simulink model "MiL_BMS_Bat"  (Simulink 7.8)
settings: Solver=ode1  SolverMode=SingleTasking  StartTime=0.0  StopTime=4000  FixedStep=0.01  RelTol=1e-3
PreLoadFcn:
  | Init_file_Bat;
values from neighbouring files (symbols this model uses):
  C_diff = 5000    [Init_file_Bat.m]
  ChargeCurrent = 5    [Init_file_Bat.m]
  ChargeSwitch = 1    [Init_file_Bat.m]
  delta_max_v_cell = 1    [Init_file_Bat.m]
  DischargeCurrent = -5    [Init_file_Bat.m]
  I_max_line = int32(10000)    [Init_file_Bat.m]
  I_min_line = int32(-10000)    [Init_file_Bat.m]
  n_cells = 12    [Init_file_Bat.m]
  poles_soc = polyfit(SoC_table, OCV_table,4)    [Init_file_Bat.m]
  Q_0 = 36000*ones(1,12)    [Init_file_Bat.m]
  R_balance = 10*ones(1,12)    [Init_file_Bat.m]
  R_ct = 3.2*10^-3    (= 0.0032)    [Init_file_Bat.m]
  R_diff = 4*10^-3    (= 0.004)    [Init_file_Bat.m]
  R_i = 2*10^-3    (= 0.002)    [Init_file_Bat.m]
  SoC_init_cells = 0.8*ones(1,12)    [Init_file_Bat.m]
  T_cells = 20*ones(1,12)    [Init_file_Bat.m]
  T_max_cell = uint16(373)    [Init_file_Bat.m]
  T_min_cell = uint16(273)    [Init_file_Bat.m]
  Ts = 10*10^-3    (= 0.01)    [Init_file_Bat.m]
  V_max_bat = uint16(49080)    [Init_file_Bat.m]
  V_max_cell = uint16(4090)    [Init_file_Bat.m]
  V_min_bat = uint16(36000)    [Init_file_Bat.m]
  V_min_cell = uint16(2800)    [Init_file_Bat.m]
undefined symbols (not defined in the file or in its folder): DiscIntNeverNeededParam, OCV_table, sigbuilder_block, SoC_table
settings Model: Creator=Schmidt  LastModifiedBy=user
settings DebuggingCC: FcnCallInpInsideContextMsg=Use local settings
settings RTWCC: SystemTargetFile=lcrt.tlc  TemplateMakefile=lcrt_default_tmf  Description=LABCAR Real-Time Target  ProcessScript=lcrt_make_rtw_hook
settings STFCustomTargetCC: ModelReferenceCompliant=off  SystemTargetFile=lcrt.tlc

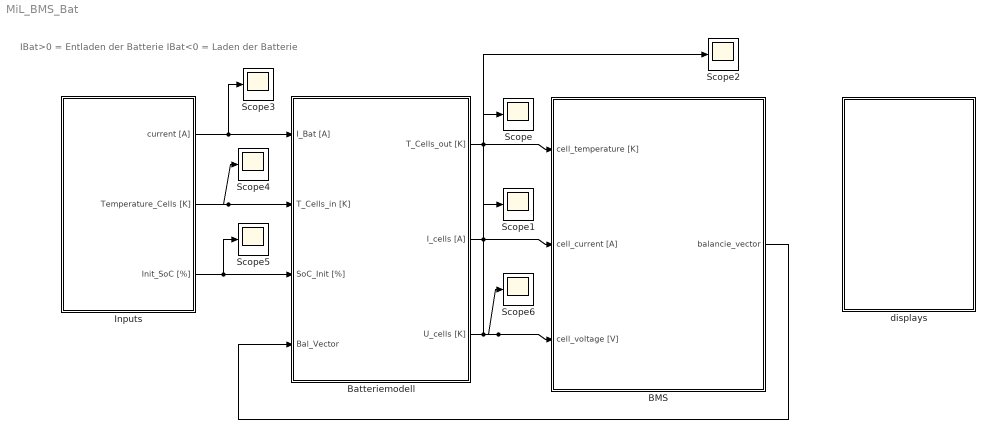
== system MiL_BMS_Bat ==
  note: IBat>0 = Entladen der Batterie
      | IBat<0 = Laden der Batterie
  BMS : Subsystem
  Batteriemodell : Subsystem
  Inputs : Subsystem
  Scope{,1..6} (7 alike) : Scope
      Scope settings: YMin=20  YMax=20  SaveName=ScopeData19
      Scope1 settings: YMin=-10  YMax=-10  SaveName=ScopeData20
      Scope2 settings: SaveName=ScopeData21
      Scope3 settings: YMin=-10  YMax=-10  SaveName=ScopeData22
      Scope4 settings: SaveName=ScopeData23
      Scope5 settings: SaveName=ScopeData24
      Scope6 settings: YMin=3.38  YMax=3.46  SaveName=ScopeData25
  displays : Subsystem
  wires:
  Batteriemodell/1(T_Cells_out [K]) -> BMS/1(cell_temperature [K]), Scope/1
  Inputs/1(current [A]) -> Batteriemodell/1(I_Bat [A]), Scope3/1
  Inputs/2(Temperature_Cells [K]) -> Batteriemodell/2(T_Cells_in [K]), Scope4/1
  Inputs/3(Init_SoC [%]) -> Batteriemodell/3(SoC_Init [%]), Scope5/1
  Batteriemodell/3(U_cells [K]) -> Scope2/1, BMS/3(cell_voltage [V]), Scope6/1
  Batteriemodell/2(I_cells [A]) -> BMS/2(cell_current [A]), Scope1/1
  BMS/1(balancie_vector) -> Batteriemodell/4(Bal_Vector)

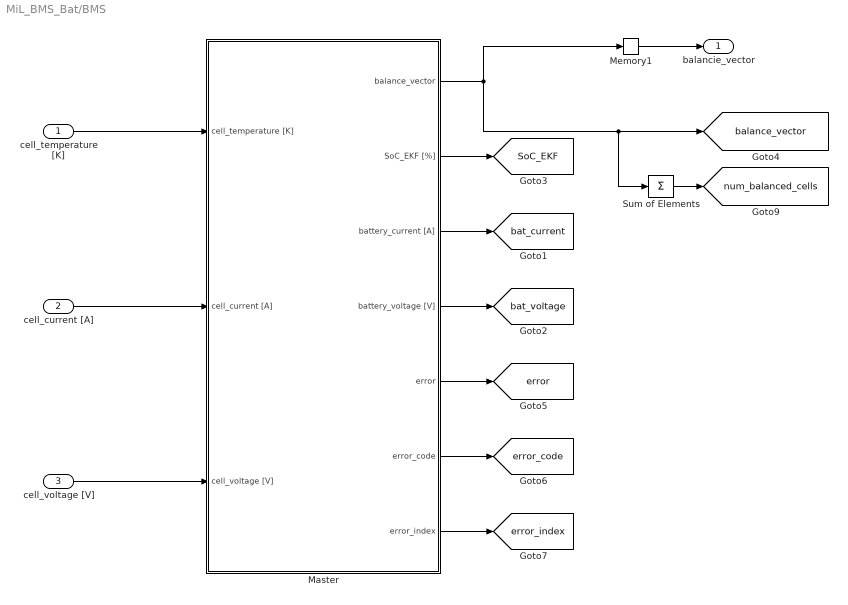
== system MiL_BMS_Bat/BMS ==
  cell_temperature [K] : Inport
  cell_current [A] : Inport  Port=2
  cell_voltage [V] : Inport  Port=3
  Master : Subsystem
  Memory1 : Memory
  Sum of Elements : Sum  Inputs=+
  balancie_vector : Outport
  tag scope: SoC_EKF=global, balance_vector=global, bat_current=global, bat_voltage=global, error=global, error_code=global, error_index=global, num_balanced_cells=global
  wires:
  Memory1/1 -> balancie_vector/1
  cell_temperature [K]/1 -> Master/1(cell_temperature [K])
  cell_voltage [V]/1 -> Master/3(cell_voltage [V])
  cell_current [A]/1 -> Master/2(cell_current [A])
  Master/2(SoC_EKF [%]) -> [SoC_EKF]
  Master/5(error) -> [error]
  Master/6(error_code) -> [error_code]
  Master/7(error_index) -> [error_index]
  Master/1(balance_vector) -> [balance_vector], Sum of Elements/1, Memory1/1
  Master/3(battery_current [A]) -> [bat_current]
  Master/4(battery_voltage [V]) -> [bat_voltage]
  Sum of Elements/1 -> [num_balanced_cells]

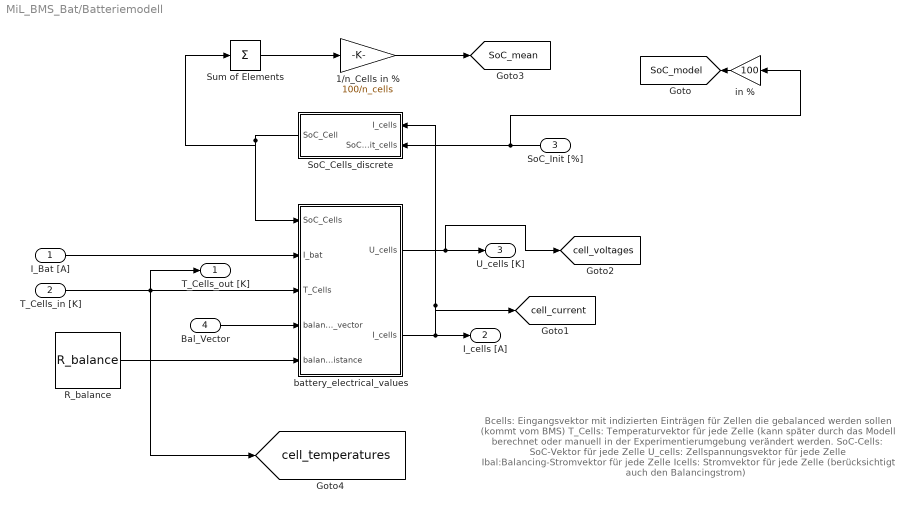
== system MiL_BMS_Bat/Batteriemodell ==
  note: Bcells: Eingangsvektor mit indizierten Einträgen
      | für Zellen die gebalanced werden sollen
      | (kommt vom BMS)
      |
      | T_Cells: Temperaturvektor für jede Zelle (kann später
      | durch das Modell berechnet oder manuell in der
      | Experimentierumgebung verändert werden.
      |
      | SoC-Cells: SoC-Vektor für jede Zelle
      |
      | U_cells: Zellspannungsvektor für jede Zelle
      |
      | Ibal:Balancing-Stromvektor für jede Zelle
      |
      | Icells: Stromvektor für jede Zelle (berücksichtigt auch
      | den Balancingstrom)
  I_Bat [A] : Inport
  T_Cells_in [K] : Inport  Port=2
  SoC_Init [%] : Inport  Port=3
  Bal_Vector : Inport  Port=4
  1/n_Cells in % : Gain  Gain=100/n_cells
  R_balance : Constant  Value=R_balance
  SoC_Cells_discrete : Subsystem
  Sum of Elements : Sum  Inputs=+
  battery_electrical_values : Subsystem
  in % : Gain  Gain=100
  T_Cells_out [K] : Outport
  I_cells [A] : Outport  Port=2
  U_cells [K] : Outport  Port=3
  tag scope: SoC_mean=global, SoC_model=global, cell_current=global, cell_temperatures=global, cell_voltages=global
  wires:
  in %/1 -> [SoC_model]
  Sum of Elements/1 -> 1/n_Cells in %/1
  1/n_Cells in %/1 -> [SoC_mean]
  SoC_Init [%]/1 -> SoC_Cells_discrete/2(SoC_init_cells), in %/1
  battery_electrical_values/2(I_cells) -> I_cells [A]/1, SoC_Cells_discrete/1(I_cells), [cell_current]
  SoC_Cells_discrete/1(SoC_Cell) -> battery_electrical_values/1(SoC_Cells), Sum of Elements/1
  T_Cells_in [K]/1 -> battery_electrical_values/3(T_Cells), T_Cells_out [K]/1, [cell_temperatures]
  I_Bat [A]/1 -> battery_electrical_values/2(I_bat)
  Bal_Vector/1 -> battery_electrical_values/4(balance_vector)
  R_balance/1 -> battery_electrical_values/5(balance_resistance)
  battery_electrical_values/1(U_cells) -> U_cells [K]/1, [cell_voltages]

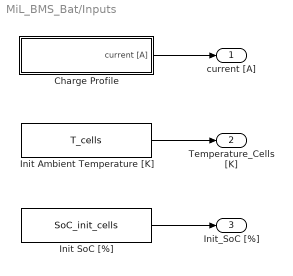
== system MiL_BMS_Bat/Inputs ==
  Charge Profile : Subsystem
  Init Ambient Temperature [K] : Constant  Value=T_cells
  Init SoC [%] : Constant  Value=SoC_init_cells
  current [A] : Outport
  Temperature_Cells [K] : Outport  Port=2
  Init_SoC [%] : Outport  Port=3
  wires:
  Charge Profile/1(current [A]) -> current [A]/1
  Init Ambient Temperature [K]/1 -> Temperature_Cells [K]/1
  Init SoC [%]/1 -> Init_SoC [%]/1

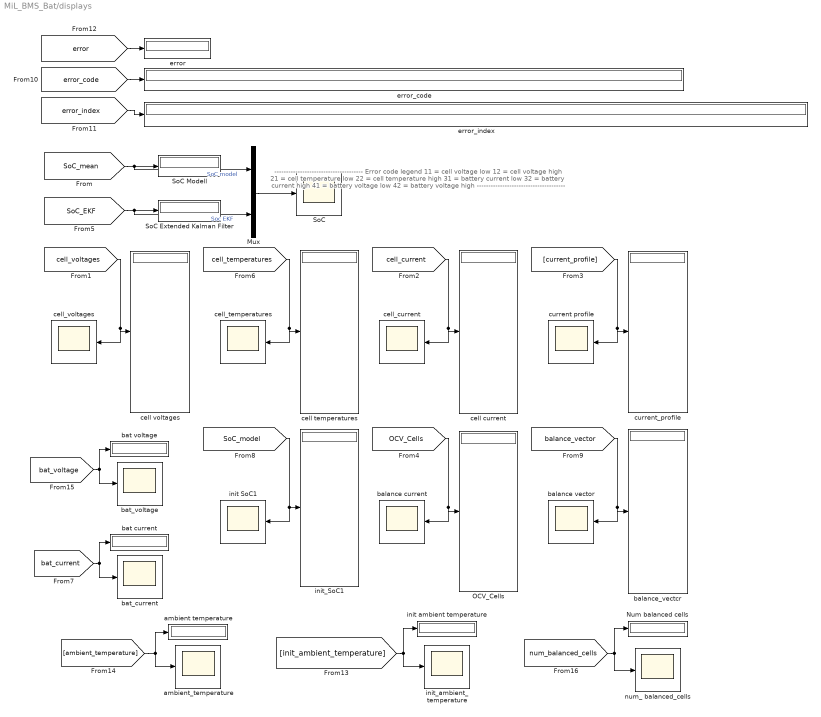
== system MiL_BMS_Bat/displays ==
  note: --------------------------------------
      | Error code legend
      | 11 = cell voltage low
      | 12 = cell voltage high
      | 21 = cell temperature low
      | 22 = cell temperature high
      | 31 = battery current low
      | 32 = battery current high
      | 41 = battery voltage low
      | 42 = battery voltage high
      | --------------------------------------
  Mux : Mux  Inputs=2
  Num balanced cells : Display
  OCV_Cells : Display
  SoC : Scope
      settings: TickLabels=on  YMin=71  YMax=74.5  SaveName=ScopeData9
  SoC Extended Kalman Filter : Display
  SoC Modell : Display
  ambient temperature : Display
  ambient_temperature : Scope
      settings: YMin=10.45  YMax=11.55
  balance current : Scope
      settings: YMin=70  YMax=80  SaveName=ScopeData16
  balance vector : Scope
      settings: YMin=70  YMax=80  SaveName=ScopeData3
  balance_vectcr : Display
  bat current : Display
  bat voltage : Display
  bat_current : Scope
      settings: YMin=0.435  YMax=0.4625  SaveName=ScopeData5
  bat_voltage : Scope
      settings: YMin=10.45  YMax=11.55  SaveName=ScopeData7
  cell current : Display
  cell temperatures : Display
  cell voltages : Display
  cell_current : Scope
      settings: YMin=70  YMax=80  SaveName=ScopeData15
  cell_temperatures : Scope
      settings: YMin=70  YMax=80  SaveName=ScopeData6
  cell_voltages : Scope
      settings: YMin=3.3675  YMax=3.36787
  current profile : Scope
      settings: YMin=70  YMax=80  SaveName=ScopeData2
  current_profile : Display
  error : Display
  error_code : Display
  error_index : Display
  init SoC1 : Scope
      settings: YMin=70  YMax=80  SaveName=ScopeData13
  init ambient temperature : Display
  init_SoC1 : Display
  init_ambient_temperature : Scope
      settings: YMin=10.45  YMax=11.55  SaveName=ScopeData17
  num_ balanced_cells : Scope
      settings: YMin=10.45  YMax=11.55  SaveName=ScopeData4
  wires:
  [cell_temperatures] -> cell temperatures/1, cell_temperatures/1
  [error_code] -> error_code/1
  [error_index] -> error_index/1
  [error] -> error/1
  [cell_voltages] -> cell voltages/1, cell_voltages/1
  [num_balanced_cells] -> Num balanced cells/1, num_ balanced_cells/1
  [SoC_EKF] -> Mux/2, SoC Extended Kalman Filter/1  "Soc EKF"
  [SoC_mean] -> SoC Modell/1, Mux/1  "SoC model"
  Mux/1 -> SoC/1
  [SoC_model] -> init_SoC1/1, init SoC1/1
  [current_profile] -> current_profile/1, current profile/1
  [cell_current] -> cell current/1, cell_current/1
  [balance_vector] -> balance_vectcr/1, balance vector/1
  [OCV_Cells] -> OCV_Cells/1, balance current/1
  [init_ambient_temperature] -> init ambient temperature/1, init_ambient_temperature/1
  [ambient_temperature] -> ambient temperature/1, ambient_temperature/1
  [bat_current] -> bat current/1, bat_current/1
  [bat_voltage] -> bat voltage/1, bat_voltage/1

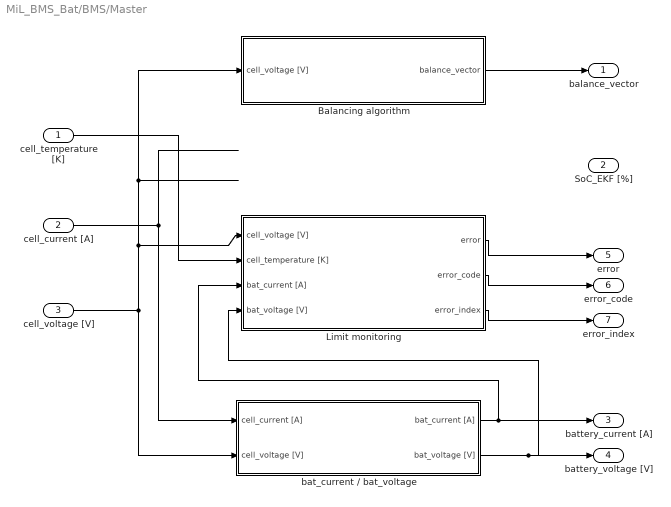
== system MiL_BMS_Bat/BMS/Master ==
  cell_temperature [K] : Inport
  cell_current [A] : Inport  Port=2
  cell_voltage [V] : Inport  Port=3
  Balancing algorithm : Subsystem
  Limit monitoring : Subsystem
  bat_current / bat_voltage : Subsystem
  balance_vector : Outport
  SoC_EKF [%] : Outport  Port=2
  battery_current [A] : Outport  Port=3
  battery_voltage [V] : Outport  Port=4
  error : Outport  Port=5
  error_code : Outport  Port=6
  error_index : Outport  Port=7
  wires:
  bat_current / bat_voltage/2(bat_voltage [V]) -> battery_voltage [V]/1, Limit monitoring/4(bat_voltage [V])
  bat_current / bat_voltage/1(bat_current [A]) -> battery_current [A]/1, Limit monitoring/3(bat_current [A])
  Balancing algorithm/1(balance_vector) -> balance_vector/1
  ? -> SoC_EKF [%]/1
  cell_voltage [V]/1 -> Balancing algorithm/1(cell_voltage [V]), Limit monitoring/1(cell_voltage [V]), bat_current / bat_voltage/2(cell_voltage [V])
  cell_current [A]/1 -> bat_current / bat_voltage/1(cell_current [A])
  cell_temperature [K]/1 -> Limit monitoring/2(cell_temperature [K])
  Limit monitoring/1(error) -> error/1
  Limit monitoring/2(error_code) -> error_code/1
  Limit monitoring/3(error_index) -> error_index/1

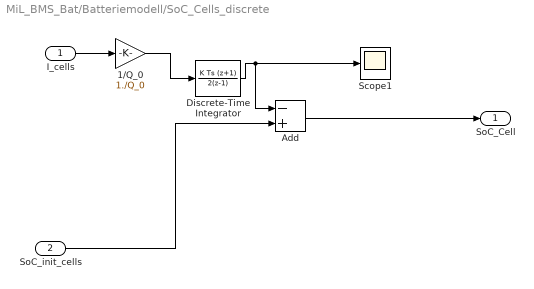
== system MiL_BMS_Bat/Batteriemodell/SoC_Cells_discrete ==
  I_cells : Inport
  SoC_init_cells : Inport  Port=2
  1/Q_0 : Gain  Gain=1./Q_0
  Add : Sum  Inputs=-+
  Discrete-Time Integrator : DiscreteIntegrator  IntegratorMethod=Integration: Trapezoidal  SampleTime=0.010  ICPrevOutput=DiscIntNeverNeededParam  ICPrevScaledInput=DiscIntNeverNeededParam
  Scope1 : Scope
      settings: SaveName=ScopeData9
  SoC_Cell : Outport
  wires:
  I_cells/1 -> 1/Q_0/1
  Add/1 -> SoC_Cell/1
  Discrete-Time Integrator/1 -> Scope1/1, Add/1
  1/Q_0/1 -> Discrete-Time Integrator/1
  SoC_init_cells/1 -> Add/2

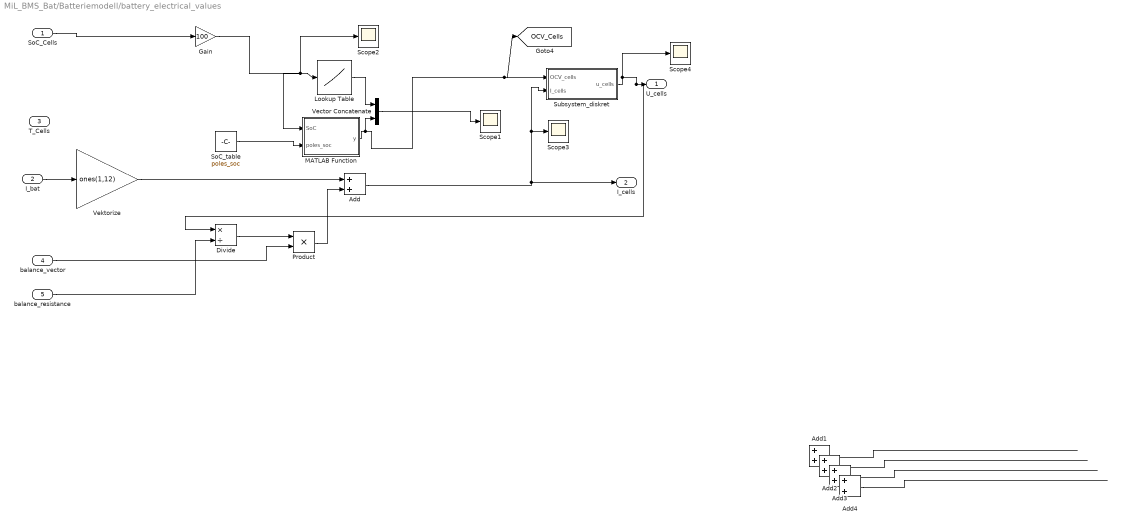
== system MiL_BMS_Bat/Batteriemodell/battery_electrical_values ==
  SoC_Cells : Inport
  I_bat : Inport  Port=2
  T_Cells : Inport  Port=3
  balance_vector : Inport  Port=4
  balance_resistance : Inport  Port=5
  " SoC_table" : Constant  Value=poles_soc
  Add{,1..4} (5 alike) : Sum
  Divide : Product  Inputs=*/
  Gain : Gain  Gain=100
  Lookup Table : Lookup  InputValues=SoC_table  Table=OCV_table  LookUpMeth=Interpolation-Use End Values  RndMeth=Round
  MATLAB Function : MATLAB Function  TreatAsAtomicUnit=on
  Product : Product  RndMeth=Zero
  Scope{1..4} (4 alike) : Scope
      Scope1 settings: YMin=3.3275  YMax=3.3575  SaveName=ScopeData4
      Scope2 settings: YMin=41  YMax=50  SaveName=ScopeData5
      Scope3 settings: SaveName=ScopeData6
      Scope4 settings: YMin=2.6  YMax=3.45  SaveName=ScopeData10
  Subsystem_diskret : Subsystem
  Vector Concatenate : Concatenate  Mode=Vector
  Vektorize : Gain  Gain=ones(1,12)
  U_cells : Outport
  I_cells : Outport  Port=2
  tag scope: OCV_Cells=global
  wires:
  SoC_Cells/1 -> Gain/1
  Subsystem_diskret/1(u_cells) -> Scope4/1, U_cells/1, Divide/1
  I_bat/1 -> Vektorize/1
  Lookup Table/1 -> Vector Concatenate/1
  Gain/1 -> Lookup Table/1, Scope2/1, MATLAB Function/1(SoC)
  Vector Concatenate/1 -> Scope1/1
  MATLAB Function/1(y) -> Vector Concatenate/2, Subsystem_diskret/1(OCV_cells), [OCV_Cells]
  " SoC_table"/1 -> MATLAB Function/2(poles_soc)
  Add1/1 -> ?
  Add2/1 -> ?
  ? -> Add2/2
  Add3/1 -> ?
  ? -> Add3/2
  Add4/1 -> ?
  ? -> Add4/2
  Divide/1 -> Product/1
  balance_vector/1 -> Product/2
  Product/1 -> Add/2
  balance_resistance/1 -> Divide/2
  Vektorize/1 -> Add/1
  Add/1 -> I_cells/1, Subsystem_diskret/2(I_cells), Scope3/1

== system MiL_BMS_Bat/Inputs/Charge Profile ==
  ChargeCurrent[A] : Constant  Value=ChargeCurrent
  ChargeCurrent[A]1 : Constant  Value=DischargeCurrent
  Constant : Constant  Value=ChargeSwitch
  Multiport Switch : MultiPortSwitch  zeroidx=off  InputSameDT=on
  virtuel drive cycle : Subsystem  Tag=STV Subsys  LoadFcn=sigbuilder_block('load');  StartFcn=sigbuilder_block('start');  StopFcn=sigbuilder_block('stop');  ClipboardFcn=sigbuilder_block('clipboard');  mask(Sigbuilder block){}
      mask help: Sigbuilder GUI
      mask init:
      | if ~strcmp(get_param(bdroot(gcbh),'SimulationStatus'),'stopped') tuvar = sigbuilder_block('maskInit'); end
      settings: CopyFcn=sigbuilder_block('copy');  DeleteFcn=sigbuilder_block('delete');  ModelCloseFcn=sigbuilder_block('modelClose');  PreSaveFcn=sigbuilder_block('preSave');  NameChangeFcn=sigbuilder_block('namechange');  OpenFcn=sigbuilder_block('open',[72.75 6 756 453 ]);  CloseFcn=sigbuilder_block('close');
      mask Display: plot(0,0,100,100,[10,10,40,40,10],[80,20,20,80,80],[40,10],[50,50], [40,27,10],[65,72,56],[40,25,25,10],[28,28,43,43]);
  current [A] : Outport
  wires:
  Multiport Switch/1 -> current [A]/1  "current[A]"
  Constant/1 -> Multiport Switch/1
  ChargeCurrent[A]1/1 -> Multiport Switch/2
  ChargeCurrent[A]/1 -> Multiport Switch/3
  virtuel drive cycle/1(Signal 1) -> Multiport Switch/4

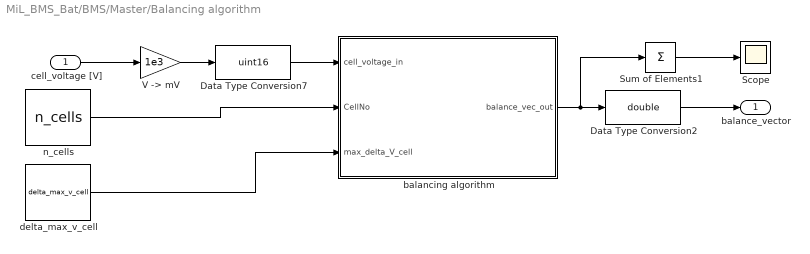
== system MiL_BMS_Bat/BMS/Master/Balancing algorithm ==
  cell_voltage [V] : Inport
  " balancing algorithm" : MATLAB Function  TreatAsAtomicUnit=on
  Data Type Conversion2 : DataTypeConversion  OutDataTypeStr=double
  Data Type Conversion7 : DataTypeConversion  OutDataTypeStr=uint16  SampleTime=Ts
  Scope : Scope
      settings: SaveName=ScopeData8
  Sum of Elements1 : Sum  Inputs=+
  "V -> mV" : Gain  Gain=1e3
  delta_max_v_cell : Constant  Value=delta_max_v_cell
  n_cells : Constant  Value=n_cells
  balance_vector : Outport
  wires:
  cell_voltage [V]/1 -> "V -> mV"/1
  " balancing algorithm"/1(balance_vec_out) -> Data Type Conversion2/1, Sum of Elements1/1
  Data Type Conversion2/1 -> balance_vector/1
  "V -> mV"/1 -> Data Type Conversion7/1
  Data Type Conversion7/1 -> " balancing algorithm"/1(cell_voltage_in)
  n_cells/1 -> " balancing algorithm"/2(CellNo)
  delta_max_v_cell/1 -> " balancing algorithm"/3(max_delta_V_cell)
  Sum of Elements1/1 -> Scope/1

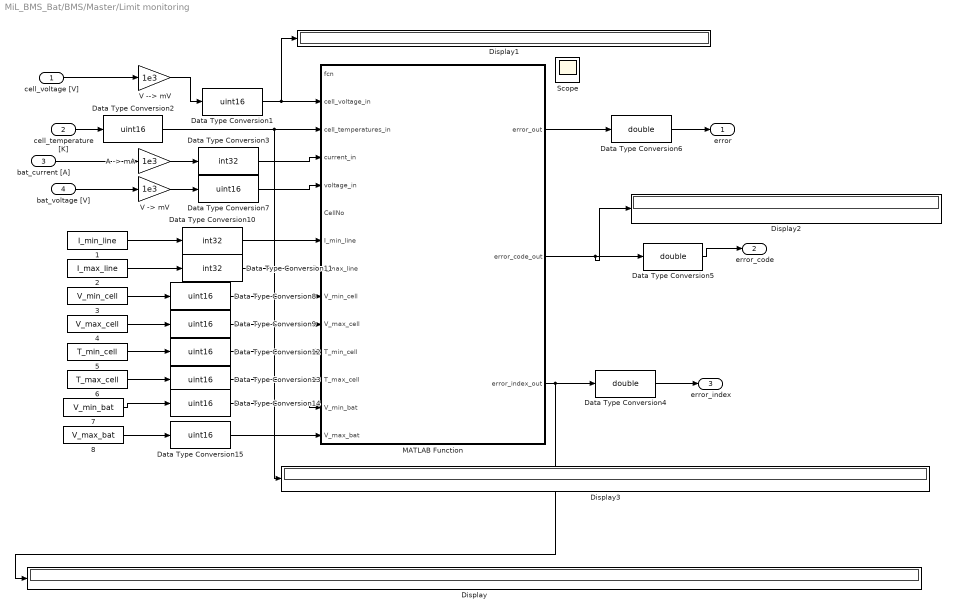
== system MiL_BMS_Bat/BMS/Master/Limit monitoring ==
  cell_voltage [V] : Inport
  cell_temperature [K] : Inport  Port=2
  bat_current [A] : Inport  Port=3
  bat_voltage [V] : Inport  Port=4
  1 : Constant  Value=I_min_line
  2 : Constant  Value=I_max_line
  3 : Constant  Value=V_min_cell
  4 : Constant  Value=V_max_cell
  5 : Constant  Value=T_min_cell
  6 : Constant  Value=T_max_cell
  7 : Constant  Value=V_min_bat
  8 : Constant  Value=V_max_bat
  "A -> mA" : Gain  Gain=1e3
  Data Type Conversion{1..2,7..9,12..15} (9 alike) : DataTypeConversion  OutDataTypeStr=uint16  SampleTime=Ts
  Data Type Conversion10 : DataTypeConversion  OutDataTypeStr=int32  SampleTime=Ts
  Data Type Conversion11 : DataTypeConversion  OutDataTypeStr=int32  SampleTime=Ts
  Data Type Conversion3 : DataTypeConversion  OutDataTypeStr=int32  SampleTime=Ts
  Data Type Conversion4 : DataTypeConversion  OutDataTypeStr=double
  Data Type Conversion5 : DataTypeConversion  OutDataTypeStr=double
  Data Type Conversion6 : DataTypeConversion  OutDataTypeStr=double
  Display{,1..3} (4 alike) : Display
  MATLAB Function : MATLAB Function  TreatAsAtomicUnit=on
  Scope : Scope
      settings: YMin=3429  YMax=3429  SaveName=ScopeData12
  V --> mV : Gain  Gain=1e3
  "V -> mV" : Gain  Gain=1e3
  error : Outport
  error_code : Outport  Port=2
  error_index : Outport  Port=3
  wires:
  Data Type Conversion6/1 -> error/1
  Data Type Conversion5/1 -> error_code/1
  "V -> mV"/1 -> Data Type Conversion7/1
  V --> mV/1 -> Data Type Conversion1/1
  "A -> mA"/1 -> Data Type Conversion3/1
  bat_current [A]/1 -> "A -> mA"/1
  cell_temperature [K]/1 -> Data Type Conversion2/1
  Data Type Conversion2/1 -> MATLAB Function/3(cell_temperatures_in), Display3/1
  Data Type Conversion3/1 -> MATLAB Function/4(current_in)
  Data Type Conversion7/1 -> MATLAB Function/5(voltage_in)
  1/1 -> Data Type Conversion10/1
  2/1 -> Data Type Conversion11/1
  3/1 -> Data Type Conversion8/1
  4/1 -> Data Type Conversion9/1
  5/1 -> Data Type Conversion12/1
  6/1 -> Data Type Conversion13/1
  7/1 -> Data Type Conversion14/1
  8/1 -> Data Type Conversion15/1
  Data Type Conversion8/1 -> MATLAB Function/9(V_min_cell)
  Data Type Conversion9/1 -> MATLAB Function/10(V_max_cell)
  Data Type Conversion10/1 -> MATLAB Function/7(I_min_line)
  Data Type Conversion11/1 -> MATLAB Function/8(I_max_line)
  Data Type Conversion12/1 -> MATLAB Function/11(T_min_cell)
  Data Type Conversion13/1 -> MATLAB Function/12(T_max_cell)
  Data Type Conversion14/1 -> MATLAB Function/13(V_min_bat)
  Data Type Conversion15/1 -> MATLAB Function/14(V_max_bat)
  Data Type Conversion1/1 -> MATLAB Function/2(cell_voltage_in), Display1/1
  MATLAB Function/1(error_out) -> Data Type Conversion6/1
  MATLAB Function/2(error_code_out) -> Data Type Conversion5/1, Display2/1
  MATLAB Function/3(error_index_out) -> Data Type Conversion4/1, Display/1
  Data Type Conversion4/1 -> error_index/1
  cell_voltage [V]/1 -> V --> mV/1
  bat_voltage [V]/1 -> "V -> mV"/1

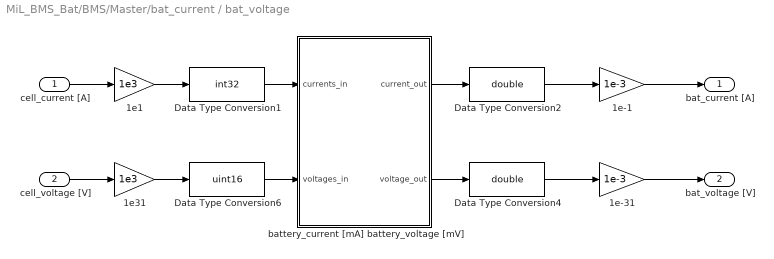
== system MiL_BMS_Bat/BMS/Master/bat_current / bat_voltage ==
  cell_current [A] : Inport
  cell_voltage [V] : Inport  Port=2
  1e-1 : Gain  Gain=1e-3
  1e-31 : Gain  Gain=1e-3
  1e1 : Gain  Gain=1e3
  1e31 : Gain  Gain=1e3
  Data Type Conversion1 : DataTypeConversion  OutDataTypeStr=int32  SampleTime=Ts
  Data Type Conversion2 : DataTypeConversion  OutDataTypeStr=double
  Data Type Conversion4 : DataTypeConversion  OutDataTypeStr=double
  Data Type Conversion6 : DataTypeConversion  OutDataTypeStr=uint16  SampleTime=Ts
  battery_current [mA] battery_voltage [mV] : MATLAB Function  TreatAsAtomicUnit=on
  bat_current [A] : Outport
  bat_voltage [V] : Outport  Port=2
  wires:
  battery_current [mA] battery_voltage [mV]/2(voltage_out) -> Data Type Conversion4/1
  battery_current [mA] battery_voltage [mV]/1(current_out) -> Data Type Conversion2/1
  1e31/1 -> Data Type Conversion6/1
  1e1/1 -> Data Type Conversion1/1
  Data Type Conversion1/1 -> battery_current [mA] battery_voltage [mV]/1(currents_in)
  cell_current [A]/1 -> 1e1/1
  Data Type Conversion6/1 -> battery_current [mA] battery_voltage [mV]/2(voltages_in)
  cell_voltage [V]/1 -> 1e31/1
  Data Type Conversion2/1 -> 1e-1/1
  1e-1/1 -> bat_current [A]/1
  Data Type Conversion4/1 -> 1e-31/1
  1e-31/1 -> bat_voltage [V]/1

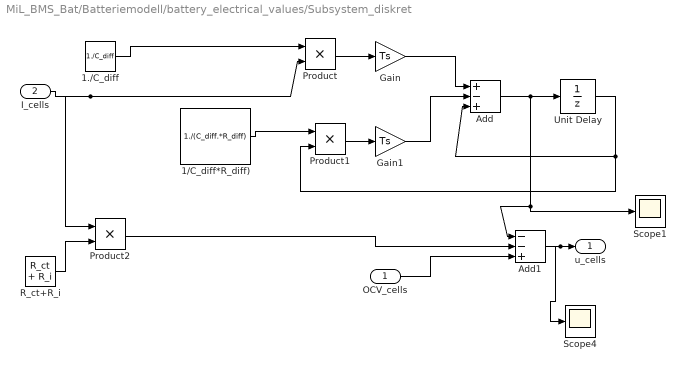
== system MiL_BMS_Bat/Batteriemodell/battery_electrical_values/Subsystem_diskret ==
  OCV_cells : Inport
  I_cells : Inport  Port=2
  1./C_diff : Constant  Value=1./C_diff
  1/C_diff*R_diff) : Constant  Value=1./(C_diff.*R_diff)
  Add : Sum  Inputs=+-+
  Add1 : Sum  Inputs=--+
  Gain : Gain  Gain=Ts
  Gain1 : Gain  Gain=Ts
  Product : Product  RndMeth=Zero
  Product1 : Product  RndMeth=Zero
  Product2 : Product  RndMeth=Zero
  R_ct+R_i : Constant  Value=R_ct + R_i
  Scope1 : Scope
      settings: TimeRange=4500  YMin=3.25  YMax=3.55  SaveName=ScopeData7
  Scope4 : Scope
      settings: TimeRange=4500  YMin=3.25  YMax=3.55  SaveName=ScopeData11
  Unit Delay : UnitDelay  SampleTime=-1
  u_cells : Outport
  wires:
  1./C_diff/1 -> Product/1
  I_cells/1 -> Product/2, Product2/1
  Gain/1 -> Add/1
  Add/1 -> Unit Delay/1, Add1/1, Scope1/1
  1/C_diff*R_diff)/1 -> Product1/1
  Unit Delay/1 -> Add/3, Product1/2
  Product1/1 -> Gain1/1
  Add1/1 -> u_cells/1, Scope4/1
  Product2/1 -> Add1/2
  OCV_cells/1 -> Add1/3
  R_ct+R_i/1 -> Product2/2
  Product/1 -> Gain/1
  Gain1/1 -> Add/2

== system MiL_BMS_Bat/Inputs/Charge Profile/virtuel drive cycle ==
  Demux : Demux  Tag=STV Demux  Outputs=1
  FromWs : FromWorkspace  Tag=STV FromWs  VariableName=tuvar  SampleTime=0  SigBuilderData=DataTag0  VnvData=DataTag1
      SigBuilderData=|
      | common.afterFinalStr = 'Extrapolate'
      | common.sampleTime = 0
      | dataSet.timeRange = [0 300]
      | dataSet.name = 'Group 1'
      | sbobj.Groups.Name = 'Group 1'
      | sbobj.Groups.Signals.Name = 'Signal 1'
      | sbobj.Groups.Signals.XData = [0 50 100 110 150 180 200 220 300]
      | sbobj.Groups.Signals.YData = [0 -2 -2.5 0.5 -1 -0.5 -2 1 -1]
      | sbobj.Groups.TimeRange = [0 300]
  Signal 1 : Outport  Tag=STV Outport
  wires:
  Demux/1 -> Signal 1/1
  FromWs/1 -> Demux/1

== matlab function BMS/Master/Balancing algorithm/ balancing algorithm ==
  data: balance_vec_out output uint8; cell_voltage_in input double; CellNo input double; max_delta_V_cell input double
function balance_vec_out  = fcn(cell_voltage_in, CellNo, max_delta_V_cell)
% balancing algorithm

temp_balance_vec=cell_voltage_in.*0;

% Output
balance_vec_out = temp_balance_vec;

== matlab function BMS/Master/bat_current / bat_voltage/battery_current [mA] battery_voltage [mV] ==
  data: current_out output double; currents_in input double; voltages_in input double; voltage_out output double
function [current_out, voltage_out]= fcn(currents_in, voltages_in)

% calculation battery voltage and battery current
voltage = uint16(sum(voltages_in)); % summation of cell voltages of a string
current = int16(mean(currents_in)); % summation of string currents


% Output
current_out = current;
voltage_out = voltage;

== matlab function BMS/Master/Limit monitoring/MATLAB Function ==
  data: fcn input double; error_out output double; cell_voltage_in input double; cell_temperatures_in input double; current_in input double; voltage_in input double; CellNo input double; I_min_line input double; I_max_line input double; V_min_cell input double; error_code_out output double; error_index_out output double; V_max_cell input double; T_min_cell input double; T_max_cell input double; V_min_bat input double; V_max_bat input double
%function [error_out, error_code_out, error_index_out] = limit_monitoring(cell_voltage_in, V_min_cell)
function [error_out, error_code_out, error_index_out] = limit_monitoring(fcn, cell_voltage_in, cell_temperatures_in, current_in, voltage_in, CellNo, I_min_line, I_max_line, V_min_cell, V_max_cell, T_min_cell, T_max_cell, V_min_bat, V_max_bat)

error_code=zeros(1,10);
index=1;
error_index=zeros(1,12);
if ( min(cell_voltage_in)<=V_min_cell ) 
   error_code(index)= uint8(11);
    index=index+1;
    %% temp_find=find(cell_voltage_in(1:12)<=V_min_cell); %%find concerning cells
   %error_index2=cell_voltage_in;
    error_index(find(cell_voltage_in <= V_min_cell))=1;
   %error_matrix(1,:)=uint8(11)*temp_find;
    %error_matrix(1,:)=uint8(11)*error_index;
end;  
if ( max(cell_voltage_in)>=V_max_cell ) 
    error_code(index) = uint8(12);
    index=index+1;
    error_index(find(cell_voltage_in>=V_max_cell))=1; %%find concerning cells
    %error_matrix(1,:)=uint8(12)*temp_find;
end;
if (min(cell_temperatures_in+273)<= T_min_cell )
    error_code(index) = uint8(21);
    index=index+1;
    error_index(find((cell_temperatures_in+273)<=T_min_cell))=1; %%find concerning cells
    %error_matrix(2,:)=uint8(21)*temp_find;
end;
if (max(cell_temperatures_in+273)>=T_max_cell )
    error_code(index) = uint8(22);
    index=index+1;
    error_index(find((cell_temperatures_in+237)>=T_max_cell))=1; %%find concerning cells
    %error_matrix(2,:)=uint8(22)*temp_find;  %%Put in error code at the place of concerning cells
end;
if (current_in>= I_max_line ) %%Charge Current to high
    error_code(index) = uint8(31);
    index=index+1;
    error_index=ones(1,length(cell_voltage_in));
    %error_matrix(3,:)=uint8(31)*ones(1,12);%%always concernes all cells
end;
if (current_in<= I_min_line ) %%Discharge current too high
    error_code(index) = uint8(32); 
    index=index+1;
error_index=ones(1,length(cell_voltage_in));
    %error_matrix(3,:)=uint8(31)*ones(1,12)
end;
if (voltage_in<= V_min_bat )
    error_code(index) = uint8(41); 
    index=index+1;
   error_index=ones(1,length(cell_voltage_in));
    %error_matrix(4,:)=uint8(41)*ones(1,12)
end;
if (voltage_in>= V_max_bat )
    error_code(index) = uint8(42); 
    index=index+1;
error_index=ones(1,length(cell_voltage_in));
    %error_matrix(4,:)=uint8(41)*ones(1,12)
end;
    
error_out=0;

error_code_out=error_code;
error_index_out=error_index;

== matlab function Batteriemodell/battery_electrical_values/MATLAB Function ==
  data: SoC input double; y output double; poles_soc input double
function y = fcn(SoC, poles_soc)
y= polyval(poles_soc, SoC);
